simulink model "DSP_TP2_1"  (R2023a)
settings: Solver=VariableStepAuto  StartTime=0.0  StopTime=10.0  RelTol=1e-3
settings Model: Creator=tanto  LastModifiedBy=tanto

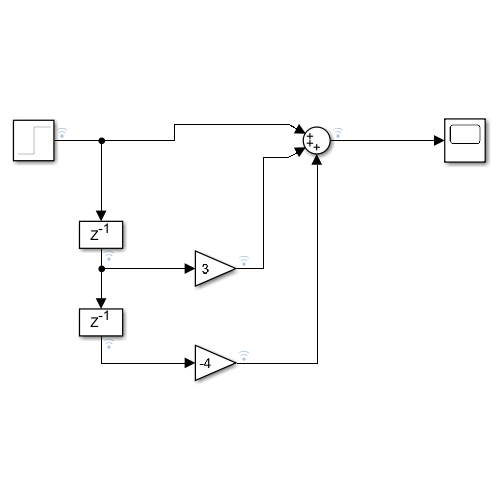
[thumbnail: Simulink's stored preview of the top-level diagram]
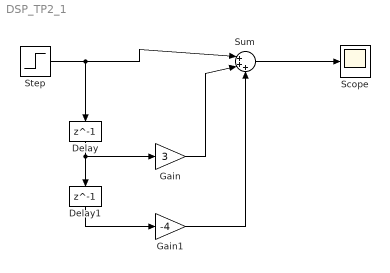
== system DSP_TP2_1 ==
  Delay : Delay  DelayLength=1  InputProcessing=Columns as channels (frame based)
  Delay1 : Delay  DelayLength=1  InputProcessing=Columns as channels (frame based)
  Gain : Gain  Gain=3
  Gain1 : Gain  Gain=-4
  Scope : Scope
  Step : Step  Time=0  SampleTime=1
  Sum : Sum  Inputs=|+++
  wires:
  Step/1 -> Sum/1, Delay/1
  Delay/1 -> Gain/1, Delay1/1
  Delay1/1 -> Gain1/1
  Gain/1 -> Sum/2
  Gain1/1 -> Sum/3
  Sum/1 -> Scope/1
